simulink model "G_p"  (Simulink 4.00)
settings: Solver=ode45  StartTime=0.0  StopTime=10.0  RelTol=1e-3
libraries: cstblocks x4
settings Model: LastModifiedBy=Administrator  BlockReductionOpt=off

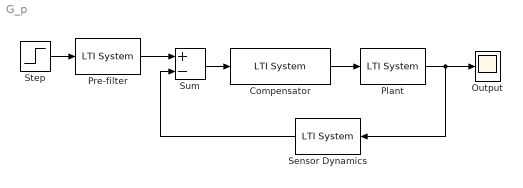
== system G_p ==
  Compensator : cstblocks/LTI System  sys=siso_tl1_regler1  IC=0
  Output : Scope
      settings: TimeRange=auto  YMin=-5  YMax=5  SaveToWorkspace=off  SaveName=ScopeData  DataFormat=Array  LimitDataPoints=on  MaxDataPoints=5000
  Plant : cstblocks/LTI System  sys=G_p  IC=0
  Pre-filter : cstblocks/LTI System  sys=F_s  IC=[]
  Sensor Dynamics : cstblocks/LTI System  Orientation=left  sys=H_s  IC=0
  Step : Step  Time=0  Before=0  After=1  SampleTime=0
  Sum : Sum  Inputs=+-  SaturateOnIntegerOverflow=on
  wires:
  Step/1 -> Pre-filter/1
  Pre-filter/1 -> Sum/1
  Sensor Dynamics/1 -> Sum/2
  Sum/1 -> Compensator/1
  Compensator/1 -> Plant/1
  Plant/1 -> Output/1, Sensor Dynamics/1
